simulink model "grid"  (R2025b)
settings: Solver=ode23t  StartTime=0.0  StopTime=0.1  RelTol=1e-3
InitFcn:
  | [P, Q, f_g, f_sw, V_dc, V_g, L_1, L_2, C_f, R_f] = lcl_param();
values from neighbouring files (symbols this model uses):
  f_g = 60    [lcl_param.m]
  f_sw = 5000    [Grid_connected_LCL_filter_code.m]    (also in LCL_filter_code.m; Load_connected_LCL_filter_code.m = 5040; Minor_Final_code.m; lcl_param.m = 15000)
  Q = 250    [lcl_param.m]
  R_f = 3*R_f    [lcl_param.m]
  V_dc = 400    [lcl_param.m]
  V_g = 120 * sqrt(3)    [lcl_param.m]
undefined symbols (not defined in the file or in its folder): PWMGenerator_2_Level__class, Three_PhaseProgrammableV_class, Three_PhaseV_IMeasuremen_class, UniversalBridge_class
libraries: fl_lib x22, nesl_utility x13, ee_lib x5, eeGeneralControl x3, slpidlib x3, eeTransforms x3, eePwmGeneratorTwoLevel x1, eeTotalHarmonicDistorsion x1, sps_lib x1
(part 2 of 2)

== system grid/LCL_Filter/Series RLC Branch9 ==
  Capacitor : fl_lib/Electrical/Electrical Elements/Capacitor  c=C_f F  r=1e-6 Ohm  g=0 1/Ohm  i_specify=off  i_priority=None  i=0 A  i_nominal_specify=off  i_nominal_value=1  i_nominal_unit=A  v_specify=off  v_priority=None  v=0 V  v_nominal_specify=off  v_nominal_value=1  v_nominal_unit=V  vc_specify=on  vc_priority=None  vc=0 V  vc_nominal_specify=off  vc_nominal_value=1  vc_nominal_unit=V
  Resistor : fl_lib/Electrical/Electrical Elements/Resistor  R=R_f Ohm  i_specify=off  i_priority=None  i=0 A  i_nominal_specify=off  i_nominal_value=1  i_nominal_unit=A  v_specify=off  v_priority=None  v=0 V  v_nominal_specify=off  v_nominal_value=1  v_nominal_unit=V
  + : PMIOPort  Side=Left
  - : PMIOPort  Port=2  Side=Right
  connections:
  Capacitor/RConn1 -- -/RConn1
  +/RConn1 -- Resistor/LConn1
  Resistor/RConn1 -- Capacitor/LConn1
